simulink model "Subsyetm"  (R2020b)
settings: Solver=VariableStepAuto  StartTime=0.0  StopTime=10.0  RelTol=1e-3
undefined symbols (not defined in the file): b, J, K, L, R
settings Model: Creator=HP  LastModifiedBy=HP

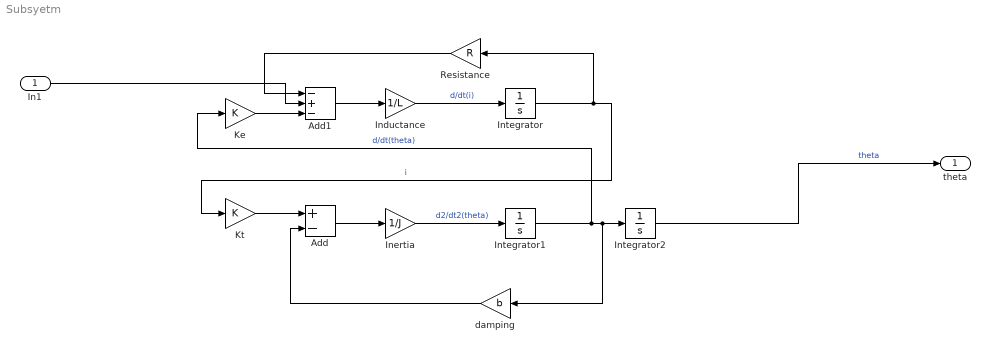
== system Subsyetm ==
  In1 : Inport  OutDataTypeStr=double  PortDimensions=1  SampleTime=0
  Add : Sum  Inputs=+-
  Add1 : Sum  Inputs=-+-
  Inductance : Gain  Gain=1/L
  Inertia : Gain  Gain=1/J
  Integrator : Integrator
  Integrator1 : Integrator
  Integrator2 : Integrator
  Ke : Gain  Gain=K
  Kt : Gain  Gain=K
  Resistance : Gain  Gain=R
  damping : Gain  Gain=b
  theta : Outport  OutDataTypeStr=double  PortDimensions=1  SampleTime=0
  wires:
  Resistance/1 -> Add1/1
  Kt/1 -> Add/1
  Add/1 -> Inertia/1
  Inertia/1 -> Integrator1/1  "d2/dt2(theta)"
  Integrator2/1 -> theta/1  "theta"
  Inductance/1 -> Integrator/1  "d/dt(i)"
  damping/1 -> Add/2
  Integrator/1 -> Resistance/1, Kt/1  "i"
  Add1/1 -> Inductance/1
  Integrator1/1 -> damping/1, Integrator2/1, Ke/1  "d/dt(theta)"
  In1/1 -> Add1/2
  Ke/1 -> Add1/3
